simulink model "acc_with_sensor"  (R2021b)
settings: Solver=FixedStepAuto  StartTime=0.0  StopTime=206  FixedStep=0.0005  RelTol=1e-3
InitFcn:
  | G=9.81;
  | m=1660;
  | rw=0.325;
  | Caf=74070;
  | Car=58525;
  | Iz=2778.5;
  | d = 1.502;
  | lf =1.1135;
  | lr =1.5065;
  | L = 2.62;
  | kph2mps=1/3.6;
values from neighbouring files (symbols this model uses):
  Leftdis_PV_switch = 2    [acc_plot_backup.m]
  s_path = [0 1.10508939428 2.2141958029 3.32141571172 4.42705301151 5.53154548532 6.63517443471 7.73808041313 8.84055018688 9.94289959674 11.0453539299 12.1480581097 ... (1001 elements, 1001x1)]    [200_100radius.mat]    (also in LV_Clothoid_S_Turn_path.mat = [0 0.966832089581 1.93621320584 2.90214024471 3.86476766313 ; NEDC_path.mat = [0 0.414605943146 0.832514087334 1.25401518562 1.68216660344; Straight_East_into_curve.mat = [0 1.65770560069 3.32192925577 4.98420060507 6.64484613518 8; acc_plot_backup.m = Station_HV_m)
  X_path = [0 1.10508939428 2.2141958029 3.32141571172 4.42705301151 5.53154548532 6.63517443471 7.73808041313 8.84055018688 9.94289959674 11.0453539299 12.1480581097 ... (1001 elements, 1001x1)]    [200_100radius.mat]    (also in LV_Clothoid_S_Turn_path.mat = [-10 -9.03316791042 -8.06378679416 -7.09785975529 -6.1352323; NEDC_path.mat = [0 0.414605943146 0.832514087334 1.25401518562 1.68216660344; Straight_East_into_curve.mat = [0 1.65770560069 3.32192925577 4.98420060507 6.64484613518 8; acc_plot_backup.m = X_HV_m)
  Y_path = [0 -1.70364610795e-18 -7.41532896709e-18 1.46822109542e-17 4.74557362791e-17 6.12980216762e-17 9.25043977736e-17 1.24088240159e-16 1.5099156923e-16 1.7058517853e-16 1.90629227614e-16 2.09673434424e-16 ... (1001 elements, 1001x1)]    [200_100radius.mat]    (also in LV_Clothoid_S_Turn_path.mat = [0 -8.46153035536e-19 5.07382551045e-18 2.07356032218e-17 3.; NEDC_path.mat = [0 -3.50680326162e-18 -2.14111304971e-18 3.38197671014e-18 3; Straight_East_into_curve.mat = [0 1.29197709199e-18 2.81882429322e-18 3.49020462564e-17 6.7; acc_plot_backup.m = Y_HV_m)
undefined symbols (not defined in the file or in its folder): C_TICK_TIME_S, Cut_in_Secenary_flg, ENUM_ACCSTATE_DISABLED, ENUM_ACCSTATE_OFF, ENUM_ACCSTATE_STANDBY, FALSE, KVDI_ACCLongPressTime_ms, KVDI_ACCMaxActSpeed_kph, KVDI_ACCSetSpdIntial_kph, KVDI_ACCSpdLargeChange_kph, KVDI_LongPressConTime_ms, ONE_FLOAT, ONE_INT, raptor_xcp_function, T, TRUE, UseTTC_switch, ZERO_FLOAT, ZERO_INT
libraries: ADASLibrary x29, simulink x22, Raptor_lib x11, dspstat3 x6, simulink_extras x6, Solver_SF x1, mpclib x1
(part 3 of 9)

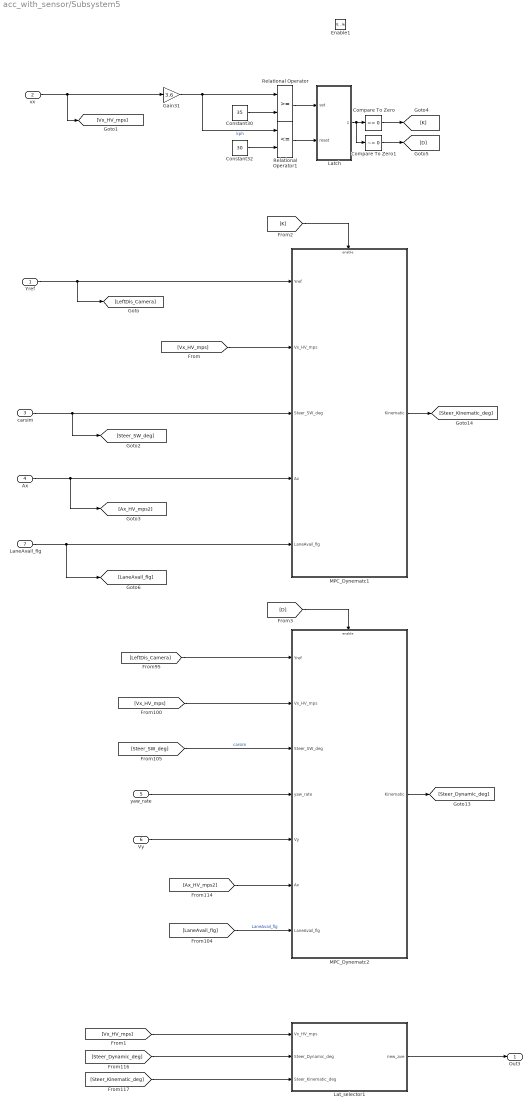
== system acc_with_sensor/Subsystem5 ==
  Yref : Inport
  vx : Inport  Port=2
  carsim : Inport  Port=3
  Ax : Inport  Port=4
  yaw_rate : Inport  Port=5
  Vy : Inport  Port=6
  LaneAvail_flg : Inport  Port=7
  Enable1 : EnablePort  StatesWhenEnabling=reset
  Compare To Zero : simulink/Logic and Bit Operations/Compare To Zero  relop===  OutDataTypeStr=boolean
  Compare To Zero1 : simulink/Logic and Bit Operations/Compare To Zero  relop=~=  OutDataTypeStr=boolean
  Constant30 : Constant  Value=35  SampleTime=-1
  Constant32 : Constant  Value=30  SampleTime=-1
  Gain31 : Gain  Gain=3.6
  Lat_selector1 : Subsystem
  Latch : Subsystem
  MPC_Dynematc1 : Subsystem
  MPC_Dynematc2 : Subsystem
  Relational Operator : RelationalOperator  OutDataTypeStr=boolean  RndMeth=Simplest
  Relational Operator1 : RelationalOperator  Operator=<=  OutDataTypeStr=boolean  RndMeth=Simplest
  Out3 : Outport
  wires:
  Yref/1 -> [LeftDis_Camera], MPC_Dynematc1/1(Yref)
  yaw_rate/1 -> MPC_Dynematc2/4(yaw_rate)
  carsim/1 -> [Steer_SW_deg], MPC_Dynematc1/3(Steer_SW_deg)
  [Steer_Dynamic_deg] -> Lat_selector1/2(Steer_Dynamic_deg)
  [Vx_HV_mps] -> MPC_Dynematc2/2(Vx_HV_mps)
  Vy/1 -> MPC_Dynematc2/5(Vy)
  Ax/1 -> [Ax_HV_mps2], MPC_Dynematc1/4(Ax)
  Lat_selector1/1(new_ave) -> Out3/1
  [Steer_Kinematic_deg] -> Lat_selector1/3(Steer_Kinematic_deg)
  MPC_Dynematc1/1(Kinematic) -> [Steer_Kinematic_deg]
  MPC_Dynematc2/1(Kinematic) -> [Steer_Dynamic_deg]
  [LeftDis_Camera] -> MPC_Dynematc2/1(Yref)
  [Steer_SW_deg] -> MPC_Dynematc2/3(Steer_SW_deg)  "carsim"
  [Ax_HV_mps2] -> MPC_Dynematc2/6(Ax)
  [Vx_HV_mps] -> Lat_selector1/1(Vx_HV_mps)
  Gain31/1 -> Relational Operator/1, Relational Operator1/1  "kph"
  Relational Operator/1 -> Latch/1(set)
  Relational Operator1/1 -> Latch/2(reset)
  Constant30/1 -> Relational Operator/2
  Constant32/1 -> Relational Operator1/2
  vx/1 -> [Vx_HV_mps], Gain31/1
  [Vx_HV_mps] -> MPC_Dynematc1/2(Vx_HV_mps)
  Latch/1(latched) -> Compare To Zero1/1, Compare To Zero/1
  Compare To Zero/1 -> [K]
  Compare To Zero1/1 -> [D]
  [K] -> MPC_Dynematc1/Enable
  [D] -> MPC_Dynematc2/Enable
  LaneAvail_flg/1 -> [LaneAvail_flg], MPC_Dynematc1/5(LaneAvail_flg)
  [LaneAvail_flg] -> MPC_Dynematc2/7(LaneAvail_flg)  "LaneAvail_flg"

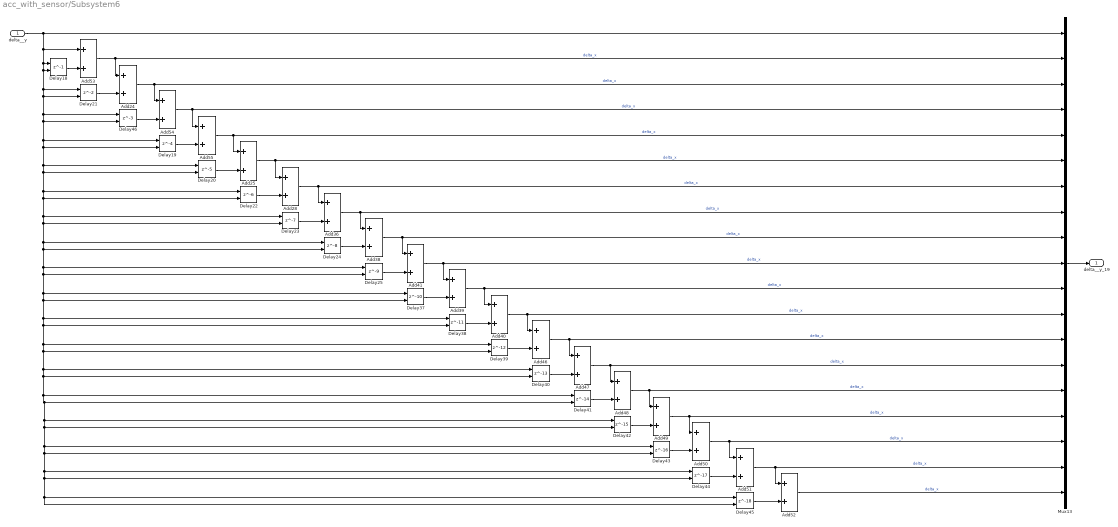
== system acc_with_sensor/Subsystem6 ==
  delta__y : Inport
  Add{24..25,28,36,38..41,46..55} (18 alike) : Sum
  Delay18 : Delay  DelayLength=1  InitialConditionSource=Input port
      settings: InputPortMap=u0,p4
  Delay19 : Delay  DelayLength=4  InitialConditionSource=Input port
      settings: InputPortMap=u0,p4
  Delay20 : Delay  DelayLength=5  InitialConditionSource=Input port
      settings: InputPortMap=u0,p4
  Delay21 : Delay  InitialConditionSource=Input port
      settings: InputPortMap=u0,p4
  Delay22 : Delay  DelayLength=6  InitialConditionSource=Input port
      settings: InputPortMap=u0,p4
  Delay23 : Delay  DelayLength=7  InitialConditionSource=Input port
      settings: InputPortMap=u0,p4
  Delay24 : Delay  DelayLength=8  InitialConditionSource=Input port
      settings: InputPortMap=u0,p4
  Delay25 : Delay  DelayLength=9  InitialConditionSource=Input port
      settings: InputPortMap=u0,p4
  Delay37 : Delay  DelayLength=10  InitialConditionSource=Input port
      settings: InputPortMap=u0,p4
  Delay38 : Delay  DelayLength=11  InitialConditionSource=Input port
      settings: InputPortMap=u0,p4
  Delay39 : Delay  DelayLength=12  InitialConditionSource=Input port
      settings: InputPortMap=u0,p4
  Delay40 : Delay  DelayLength=13  InitialConditionSource=Input port
      settings: InputPortMap=u0,p4
  Delay41 : Delay  DelayLength=14  InitialConditionSource=Input port
      settings: InputPortMap=u0,p4
  Delay42 : Delay  DelayLength=15  InitialConditionSource=Input port
      settings: InputPortMap=u0,p4
  Delay43 : Delay  DelayLength=16  InitialConditionSource=Input port
      settings: InputPortMap=u0,p4
  Delay44 : Delay  DelayLength=17  InitialConditionSource=Input port
      settings: InputPortMap=u0,p4
  Delay45 : Delay  DelayLength=18  InitialConditionSource=Input port
      settings: InputPortMap=u0,p4
  Delay46 : Delay  DelayLength=3  InitialConditionSource=Input port
      settings: InputPortMap=u0,p4
  Mux13 : Mux  Inputs=19
  delta__y_19 : Outport
  wires:
  Delay21/1 -> Add24/2
  delta__y/1 -> Mux13/1, Delay21/2, Delay46/1, Delay22/1, Delay25/2, Delay37/1, Delay39/2, Delay40/1, Delay41/1, Delay42/1, Delay42/2, Delay43/1, Delay44/1, Delay45/1, Delay45/2, Delay44/2, Delay43/2, Delay41/2, Delay40/2, Delay39/1, Delay38/2, Delay38/1, Delay37/2, Delay25/1, Delay24/2, Delay24/1, Delay23/2, Delay23/1, Delay22/2, Delay20/2, Delay20/1, Delay19/2, Delay19/1, Delay46/2, Delay21/1, Delay18/2, Delay18/1, Add53/1
  Delay22/1 -> Add28/2
  Add46/1 -> Mux13/13, Add47/1  "delta_x"
  Delay37/1 -> Add39/2
  Add39/1 -> Mux13/11, Add40/1  "delta_x"
  Delay38/1 -> Add40/2
  Add40/1 -> Mux13/12, Add46/1  "delta_x"
  Add38/1 -> Mux13/9, Add41/1  "delta_x"
  Add53/1 -> Mux13/2, Add24/1  "delta_x"
  Add55/1 -> Mux13/5, Add25/1  "delta_x"
  Add50/1 -> Add51/1, Mux13/17  "delta_x"
  Add47/1 -> Mux13/14, Add48/1  "delta_x"
  Delay39/1 -> Add46/2
  Delay40/1 -> Add47/2
  Mux13/1 -> delta__y_19/1
  Delay46/1 -> Add54/2
  Delay25/1 -> Add41/2
  Add52/1 -> Mux13/19  "delta_x"
  Add28/1 -> Mux13/7, Add36/1  "delta_x"
  Add36/1 -> Mux13/8, Add38/1  "delta_x"
  Delay23/1 -> Add36/2
  Delay20/1 -> Add25/2
  Delay42/1 -> Add49/2
  Delay44/1 -> Add51/2
  Delay18/1 -> Add53/2
  Add25/1 -> Mux13/6, Add28/1  "delta_x"
  Add41/1 -> Mux13/10, Add39/1  "delta_x"
  Add49/1 -> Add50/1, Mux13/16  "delta_x"
  Add51/1 -> Add52/1, Mux13/18  "delta_x"
  Delay19/1 -> Add55/2
  Add24/1 -> Mux13/3, Add54/1  "delta_x"
  Delay45/1 -> Add52/2
  Delay41/1 -> Add48/2
  Add54/1 -> Mux13/4, Add55/1  "delta_x"
  Delay24/1 -> Add38/2
  Delay43/1 -> Add50/2
  Add48/1 -> Mux13/15, Add49/1  "delta_x"

== system acc_with_sensor/Subsystem7 ==
  A : Inport
  B : Inport  Port=2
  C : Inport  Port=3
  Yref : Inport  Port=4
  x_state : Inport  Port=5
  u_old : Inport  Port=6
  Enable : EnablePort  StatesWhenEnabling=reset
  Constant104 : Constant  Value=Np  SampleTime=T
  Constant105 : Constant  Value=Nc  SampleTime=T
  Constant106 : Constant  Value=Q  SampleTime=T
  Constant107 : Constant  Value=R  SampleTime=T
  MPC_ACC4 : MATLAB Function  TreatAsAtomicUnit=on
  cmd : Outport
  wires:
  u_old/1 -> MPC_ACC4/10(u_old)
  Constant107/1 -> MPC_ACC4/9(Rs)
  Constant104/1 -> MPC_ACC4/6(Np)
  Constant106/1 -> MPC_ACC4/8(Qs)
  MPC_ACC4/1(u) -> cmd/1  "cmd"
  Constant105/1 -> MPC_ACC4/7(Nc)
  A/1 -> MPC_ACC4/1(A)
  C/1 -> MPC_ACC4/3(C)
  Yref/1 -> MPC_ACC4/4(Yref)
  B/1 -> MPC_ACC4/2(B)
  x_state/1 -> MPC_ACC4/5(x_state)

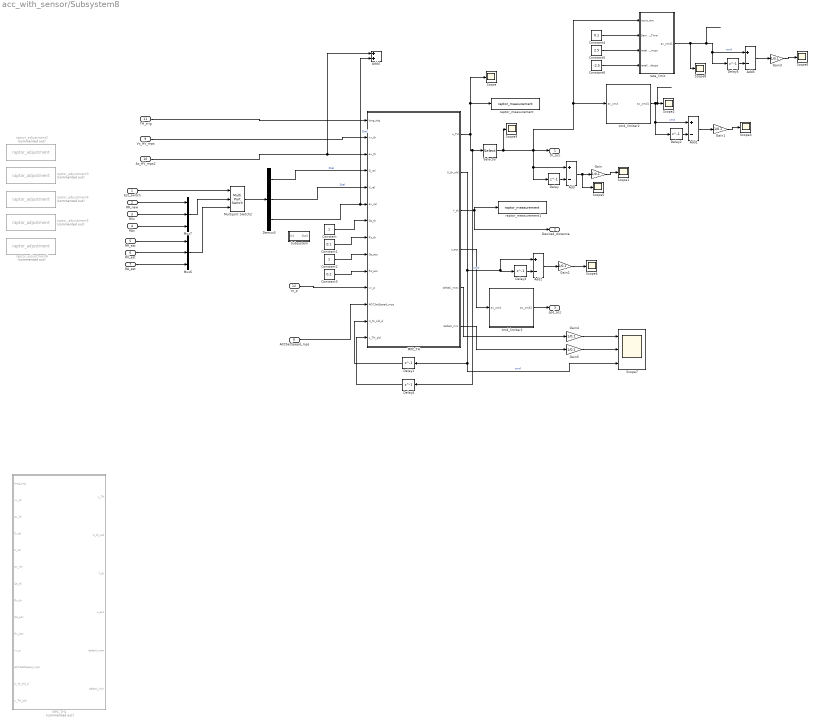
== system acc_with_sensor/Subsystem8 ==
  Est_switch : Inport
  RR_new : Inport  Port=2
  RVx : Inport  Port=3
  RAx : Inport  Port=4
  RR_est : Inport  Port=5
  RV_est : Inport  Port=6
  RA_est : Inport  Port=7
  ACCSetSpeed_mps : Inport  Port=8
  Vx_HV_mps : Inport  Port=9
  Ax_HV_mps2 : Inport  Port=10
  TH_trig : Inport  Port=11
  vx_p : Inport  Port=12
  Add{,1..3} (4 alike) : Sum  Inputs=+-
  Add4 : Sum
  Constant : Constant  SampleTime=T
  Constant1 : Constant  Value=0.1  SampleTime=T
  Constant2 : Constant  SampleTime=T
  Constant3 : Constant  Value=0.2  SampleTime=T
  Constant4 : Constant  Value=0.1  SampleTime=T
  Constant5 : Constant  Value=2.5  SampleTime=T
  Constant6 : Constant  Value=-2.5  SampleTime=T
  Delay{,2..3,5} (4 alike) : Delay  DelayLength=1
  Delay1 : Delay  DelayLength=1  SampleTime=T
  Delay4 : Delay  DelayLength=1  SampleTime=T
  Demux3 : Demux  Outputs=3
  Gain{,1..5} (6 alike) : Gain  Gain=1/0.1
  MPC_TH : MATLAB Function  TreatAsAtomicUnit=on
  MPC_TH1 : MATLAB Function  Commented=on  TreatAsAtomicUnit=on
  Multiport Switch2 : MultiPortSwitch  DataPortOrder=Zero-based contiguous  Inputs=2  DiagnosticForDefault=None  zeroidx=on
  Mux6 : Mux  Inputs=3
  Mux7 : Mux  Inputs=3
  Scope{,1..6,8..9} (9 alike) : Scope
  Scope7 : Scope  NumInputPorts=3
  Selector : Selector  InputPortWidth=3  IndexOptions=Index vector (dialog)  Indices=[1]  OutputSizes=1
  Subsystem : Subsystem
  cmd_limiter1 : Subsystem
  cmd_limiter2 : Subsystem
  raptor_adjustment2 : Raptor_lib/Data Storage/raptor_adjustment  Commented=on  paramName='Vx_th'  nameSource=Parameter  initValue=0.00  dataType=double  storage=Calibration  calDispType=Number  calEnum={'False', 'True'}  calGain=1.0  calOffset=0.0  calMax=inf  calMin=-inf  calFormat='-1'  calUnit=''  calHelp=''  calAccess=1  calFunction=raptor_xcp_function(gcb)  calDispHeaders=off  calColHeaders={'Col1' 'Col2' 'Col3'}  calRowHeaders={'Row1' 'Row2' 'Row3'}
      settings: SourceProductName=Raptor
  raptor_adjustment3 : Raptor_lib/Data Storage/raptor_adjustment  Commented=on  paramName='Ax_th'  nameSource=Parameter  initValue=0.00  dataType=double  storage=Calibration  calDispType=Number  calEnum={'False', 'True'}  calGain=1.0  calOffset=0.0  calMax=inf  calMin=-inf  calFormat='-1'  calUnit=''  calHelp=''  calAccess=1  calFunction=raptor_xcp_function(gcb)  calDispHeaders=off  calColHeaders={'Col1' 'Col2' 'Col3'}  calRowHeaders={'Row1' 'Row2' 'Row3'}
      settings: SourceProductName=Raptor
  raptor_adjustment4 : Raptor_lib/Data Storage/raptor_adjustment  Commented=on  paramName='D_rel'  nameSource=Parameter  initValue=1  dataType=double  storage=Calibration  calDispType=Number  calEnum={'False', 'True'}  calGain=1.0  calOffset=0.0  calMax=inf  calMin=-inf  calFormat='-1'  calUnit=''  calHelp=''  calAccess=1  calFunction=raptor_xcp_function(gcb)  calDispHeaders=off  calColHeaders={'Col1' 'Col2' 'Col3'}  calRowHeaders={'Row1' 'Row2' 'Row3'}
      settings: SourceProductName=Raptor
  raptor_adjustment5 : Raptor_lib/Data Storage/raptor_adjustment  Commented=on  paramName='V_rel'  nameSource=Parameter  initValue=1  dataType=double  storage=Calibration  calDispType=Number  calEnum={'False', 'True'}  calGain=1.0  calOffset=0.0  calMax=inf  calMin=-inf  calFormat='-1'  calUnit=''  calHelp=''  calAccess=1  calFunction=raptor_xcp_function(gcb)  calDispHeaders=off  calColHeaders={'Col1' 'Col2' 'Col3'}  calRowHeaders={'Row1' 'Row2' 'Row3'}
      settings: SourceProductName=Raptor
  raptor_adjustment6 : Raptor_lib/Data Storage/raptor_adjustment  Commented=on  paramName='ax_rel'  nameSource=Parameter  initValue=1  dataType=double  storage=Calibration  calDispType=Number  calEnum={'False', 'True'}  calGain=1.0  calOffset=0.0  calMax=inf  calMin=-inf  calFormat='-1'  calUnit=''  calHelp=''  calAccess=1  calFunction=raptor_xcp_function(gcb)  calDispHeaders=off  calColHeaders={'Col1' 'Col2' 'Col3'}  calRowHeaders={'Row1' 'Row2' 'Row3'}
      settings: SourceProductName=Raptor
  raptor_measurement : Raptor_lib/Data Storage/raptor_measurement  paramName='TH_acc'  nameSource=Parameter  calDispType=Number  calEnum={'False', 'True'}  calGain=1.0  calOffset=0.0  calMax=inf  calMin=-inf  calFormat='-1'  calUnit=''  calHelp=''  calAccess=1  calFunction=raptor_xcp_function(gcb)  calVisible=on
      settings: SourceProductName=Raptor
  raptor_measurement1 : Raptor_lib/Data Storage/raptor_measurement  paramName='Desired_distance'  nameSource=Parameter  calDispType=Number  calEnum={'False', 'True'}  calGain=1.0  calOffset=0.0  calMax=inf  calMin=-inf  calFormat='-1'  calUnit=''  calHelp=''  calAccess=1  calFunction=raptor_xcp_function(gcb)  calVisible=on
      settings: SourceProductName=Raptor
  rate_limit : Subsystem
  th_acc : Outport
  Desired_distance : Outport  Port=2
  spd_acc : Outport  Port=3
  wires:
  Demux3/3 -> Add4/2, MPC_TH/6(ax_rel)  "Drel"
  Demux3/2 -> MPC_TH/5(V_rel)  "Drel"
  ACCSetSpeed_mps/1 -> MPC_TH/12(ACCSetSpeed_mps)
  Est_switch/1 -> Multiport Switch2/1
  RA_est/1 -> Mux6/3
  RVx/1 -> Mux7/2
  Constant/1 -> MPC_TH/7(Qs_th)
  Vx_HV_mps/1 -> MPC_TH/2(vx_th)
  MPC_TH/3(Y_th) -> Desired_distance/1, raptor_measurement1/1
  Mux6/1 -> Multiport Switch2/3
  Mux7/1 -> Multiport Switch2/2
  Ax_HV_mps2/1 -> Add4/1, MPC_TH/3(ax_th)
  RAx/1 -> Mux7/3
  RR_est/1 -> Mux6/1
  Constant1/1 -> MPC_TH/8(Rs_th)
  Demux3/1 -> MPC_TH/4(D_rel)  "Drel"
  TH_trig/1 -> MPC_TH/1(long_trig)
  RR_new/1 -> Mux7/1
  RV_est/1 -> Mux6/2
  MPC_TH/1(u_TH) -> Delay4/1, Selector/1, raptor_measurement/1, Scope/1  "cmd"
  Multiport Switch2/1 -> Demux3/1
  Constant2/1 -> MPC_TH/9(Qs_acc)
  Constant3/1 -> MPC_TH/10(Rs_acc)
  MPC_TH/4(u_acc) -> cmd_limiter1/1(ax_cmd)
  cmd_limiter1/1(ax_cmd1) -> spd_acc/1
  vx_p/1 -> MPC_TH/11(vx_p)
  Delay/1 -> Add/2
  Add/1 -> Scope5/1, Gain/1
  Gain/1 -> Scope1/1
  Delay1/1 -> MPC_TH/13(U_th_old_d)
  Gain1/1 -> Scope3/1
  Add1/1 -> Gain1/1
  Delay2/1 -> Add1/2
  cmd_limiter2/1(ax_cmd1) -> Add1/1, Delay2/1, Scope2/1  "cmd"
  Gain2/1 -> Scope4/1
  Add2/1 -> Gain2/1
  Delay3/1 -> Add2/2
  MPC_TH/2(U_th_old) -> Add2/1, Delay3/1, Delay1/1, Scope7/3  "cmd"
  Delay4/1 -> MPC_TH/14(u_TH_old)
  Constant5/1 -> rate_limit/3(ratelimt_incps)
  Constant4/1 -> rate_limit/2(Sample_Time)
  Constant6/1 -> rate_limit/4(ratelimt_decps)
  rate_limit/1(ax_cmd1) -> Scope8/1, Delay5/1, Add3/1  "cmd"
  Delay5/1 -> Add3/2
  Add3/1 -> Gain3/1
  Gain3/1 -> Scope6/1
  MPC_TH/5(deltaU_max) -> Gain4/1
  MPC_TH/6(deltaU_min) -> Gain5/1
  Gain4/1 -> Scope7/1
  Gain5/1 -> Scope7/2
  Selector/1 -> Scope9/1, th_acc/1, rate_limit/1(input_raw), cmd_limiter2/1(ax_cmd), Delay/1, Add/1

== system acc_with_sensor/V_rel Estimation ==
  cut_in_flg : Inport
  a_c : Inport  Port=2
  S_rel : Inport  Port=3
  initial_value : Inport  Port=4
  Enable : EnablePort  StatesWhenEnabling=reset
  Add3 : Sum  Inputs=-+
  Delay1 : Delay  DelayLength=1  InitialConditionSource=Input port  SampleTime=T
      settings: InputPortMap=u0,p4
  Kalman filter : Subsystem
  sample time : Gain  Gain=1/0.1
  s_rel : Outport
  v_rel : Outport  Port=2
  a_rel : Outport  Port=3
  wires:
  S_rel/1 -> Kalman filter/3(S_rel)
  Kalman filter/1(s_rel) -> s_rel/1
  Add3/1 -> sample time/1
  Delay1/1 -> Add3/1
  a_c/1 -> Delay1/1, Delay1/2, Add3/2
  Kalman filter/2(v_rel) -> v_rel/1
  sample time/1 -> Kalman filter/2(Jerk)  "Jerk"
  Kalman filter/3(a_rel) -> a_rel/1
  initial_value/1 -> Kalman filter/4(initial_value)
  cut_in_flg/1 -> Kalman filter/1(cut_in_flg)

== system acc_with_sensor/cmd_limiter1 ==
  ax_cmd : Inport
  Constant : Constant  Value=0.1  SampleTime=T
  Constant1 : Constant  Value=2.5  SampleTime=T
  Constant2 : Constant  Value=-2.5  SampleTime=T
  Saturation : Saturate  UpperLimit=2  LowerLimit=-2
  rate_limit : Subsystem
  ax_cmd1 : Outport
  wires:
  Saturation/1 -> rate_limit/1(input_raw)
  Constant2/1 -> rate_limit/4(ratelimt_decps)
  Constant1/1 -> rate_limit/3(ratelimt_incps)
  ax_cmd/1 -> Saturation/1
  Constant/1 -> rate_limit/2(Sample_Time)
  rate_limit/1(ax_cmd1) -> ax_cmd1/1

== system acc_with_sensor/cmd_limiter11 ==
  ax_cmd : Inport
  Constant : Constant  Value=0.1  SampleTime=T
  Constant1 : Constant  Value=2.5  SampleTime=T
  Constant2 : Constant  Value=-2.5  SampleTime=T
  Constant3 : Constant  Value=2  SampleTime=T
  Constant4 : Constant  Value=-2  SampleTime=T
  Limit : ADASLibrary/Limit  SystemSampleTime=-1  VariantActivationTime=update diagram  Latency=0  AutoFrameSizeCalculation=off
      settings: SourceProductName=ADASLibrary
  rate_limit : Subsystem
  ax_cmd1 : Outport
  wires:
  rate_limit/1(ax_cmd1) -> ax_cmd1/1
  Constant/1 -> rate_limit/2(Sample_Time)
  ax_cmd/1 -> Limit/1
  Constant1/1 -> rate_limit/3(ratelimt_incps)
  Constant2/1 -> rate_limit/4(ratelimt_decps)
  Limit/1 -> rate_limit/1(input_raw)
  Constant3/1 -> Limit/2
  Constant4/1 -> Limit/3

== system acc_with_sensor/cmd_limiter2 ==
  ax_cmd : Inport
  Constant : Constant  Value=0.1  SampleTime=T
  Constant1 : Constant  Value=2.5  SampleTime=T
  Constant2 : Constant  Value=-2.5  SampleTime=T
  Constant3 : Constant  Value=2  SampleTime=T
  Constant4 : Constant  Value=-2  SampleTime=T
  Limit : ADASLibrary/Limit  SystemSampleTime=-1  VariantActivationTime=update diagram  Latency=0  AutoFrameSizeCalculation=off
      settings: SourceProductName=ADASLibrary
  rate_limit : Subsystem
  ax_cmd1 : Outport
  wires:
  Constant4/1 -> Limit/3
  Constant3/1 -> Limit/2
  Limit/1 -> rate_limit/1(input_raw)
  Constant2/1 -> rate_limit/4(ratelimt_decps)
  Constant1/1 -> rate_limit/3(ratelimt_incps)
  ax_cmd/1 -> Limit/1
  Constant/1 -> rate_limit/2(Sample_Time)
  rate_limit/1(ax_cmd1) -> ax_cmd1/1

== system acc_with_sensor/cmd_limiter3 ==
  ax_cmd : Inport
  Constant : Constant  Value=0.1  SampleTime=T
  Constant1 : Constant  Value=2.5  SampleTime=T
  Constant2 : Constant  Value=-2.5  SampleTime=T
  Constant3 : Constant  Value=2  SampleTime=T
  Constant4 : Constant  Value=-2  SampleTime=T
  Limit : ADASLibrary/Limit  SystemSampleTime=-1  VariantActivationTime=update diagram  Latency=0  AutoFrameSizeCalculation=off
      settings: SourceProductName=ADASLibrary
  rate_limit : Subsystem
  ax_cmd1 : Outport
  wires:
  Constant4/1 -> Limit/3
  Constant3/1 -> Limit/2
  Limit/1 -> rate_limit/1(input_raw)
  Constant2/1 -> rate_limit/4(ratelimt_decps)
  Constant1/1 -> rate_limit/3(ratelimt_incps)
  ax_cmd/1 -> Limit/1
  Constant/1 -> rate_limit/2(Sample_Time)
  rate_limit/1(ax_cmd1) -> ax_cmd1/1

== system acc_with_sensor/cmd_limiter4 ==
  ax_cmd : Inport
  Constant : Constant  Value=0.1  SampleTime=T
  Constant1 : Constant  Value=2.5  SampleTime=T
  Constant2 : Constant  Value=-2.5  SampleTime=T
  Saturation : Saturate  UpperLimit=2  LowerLimit=-2
  rate_limit : Subsystem
  ax_cmd1 : Outport
  wires:
  rate_limit/1(ax_cmd1) -> ax_cmd1/1
  Constant/1 -> rate_limit/2(Sample_Time)
  ax_cmd/1 -> Saturation/1
  Constant1/1 -> rate_limit/3(ratelimt_incps)
  Constant2/1 -> rate_limit/4(ratelimt_decps)
  Saturation/1 -> rate_limit/1(input_raw)

== system acc_with_sensor/cmd_limiter9 ==
  ax_cmd : Inport
  Constant : Constant  Value=0.1  SampleTime=T
  Constant1 : Constant  Value=2.5  SampleTime=T
  Constant2 : Constant  Value=-2.5  SampleTime=T
  Saturation : Saturate  UpperLimit=2  LowerLimit=-2
  rate_limit : Subsystem
  ax_cmd1 : Outport
  wires:
  rate_limit/1(ax_cmd1) -> ax_cmd1/1
  Constant/1 -> rate_limit/2(Sample_Time)
  ax_cmd/1 -> Saturation/1
  Constant1/1 -> rate_limit/3(ratelimt_incps)
  Constant2/1 -> rate_limit/4(ratelimt_decps)
  Saturation/1 -> rate_limit/1(input_raw)

== system acc_with_sensor/divide ==
  dividend : Inport
  divisor : Inport  Port=2
  default_value : Inport  Port=3
  Divide : Product  Inputs=*/
  Interval Test : simulink/Logic and Bit Operations/Interval Test  IntervalClosedRight=on  uplimit=5/3.6  IntervalClosedLeft=on  lowlimit=-1  OutDataTypeStr=boolean
  Logical Operator : Logic  Operator=NOT  Inputs=1  AllPortsSameDT=off  OutDataTypeStr=boolean
  Scope : Scope
  Switch : Switch  Criteria=u2 ~= 0  Threshold=0.5
  quotient : Outport
  wires:
  Logical Operator/1 -> Switch/2
  default_value/1 -> Switch/3  "default_value"
  Interval Test/1 -> Scope/1, Logical Operator/1
  Switch/1 -> quotient/1
  Divide/1 -> Switch/1
  divisor/1 -> Interval Test/1, Divide/2  "divisor"
  dividend/1 -> Divide/1  "dividend"

== system acc_with_sensor/divide2 ==
  dividend : Inport
  divisor : Inport  Port=2
  default_value : Inport  Port=3
  Divide : Product  Inputs=*/
  Interval Test : simulink/Logic and Bit Operations/Interval Test  IntervalClosedRight=on  uplimit=15/3.6  IntervalClosedLeft=on  lowlimit=-1  OutDataTypeStr=boolean
  Logical Operator : Logic  Operator=NOT  Inputs=1  AllPortsSameDT=off  OutDataTypeStr=boolean
  Scope : Scope
  Switch : Switch  Criteria=u2 ~= 0  Threshold=0.5
  quotient : Outport
  wires:
  dividend/1 -> Divide/1  "dividend"
  divisor/1 -> Divide/2, Interval Test/1  "divisor"
  Divide/1 -> Switch/1
  Switch/1 -> quotient/1
  Interval Test/1 -> Logical Operator/1, Scope/1
  default_value/1 -> Switch/3  "default_value"
  Logical Operator/1 -> Switch/2

== system acc_with_sensor/divide3 ==
  dividend : Inport
  divisor : Inport  Port=2
  default_value : Inport  Port=3
  Divide : Product  Inputs=*/
  Interval Test : simulink/Logic and Bit Operations/Interval Test  IntervalClosedRight=on  uplimit=-0.1  IntervalClosedLeft=on  lowlimit=-inf  OutDataTypeStr=boolean
  Logical Operator : Logic  Operator=NOT  Inputs=1  AllPortsSameDT=off  OutDataTypeStr=boolean
  Scope : Scope
  Switch : Switch  Criteria=u2 ~= 0  Threshold=0.5
  quotient : Outport
  wires:
  dividend/1 -> Divide/1  "dividend"
  divisor/1 -> Divide/2, Interval Test/1  "divisor"
  Divide/1 -> Switch/1
  Switch/1 -> quotient/1
  Interval Test/1 -> Logical Operator/1, Scope/1
  default_value/1 -> Switch/3  "default_value"
  Logical Operator/1 -> Switch/2

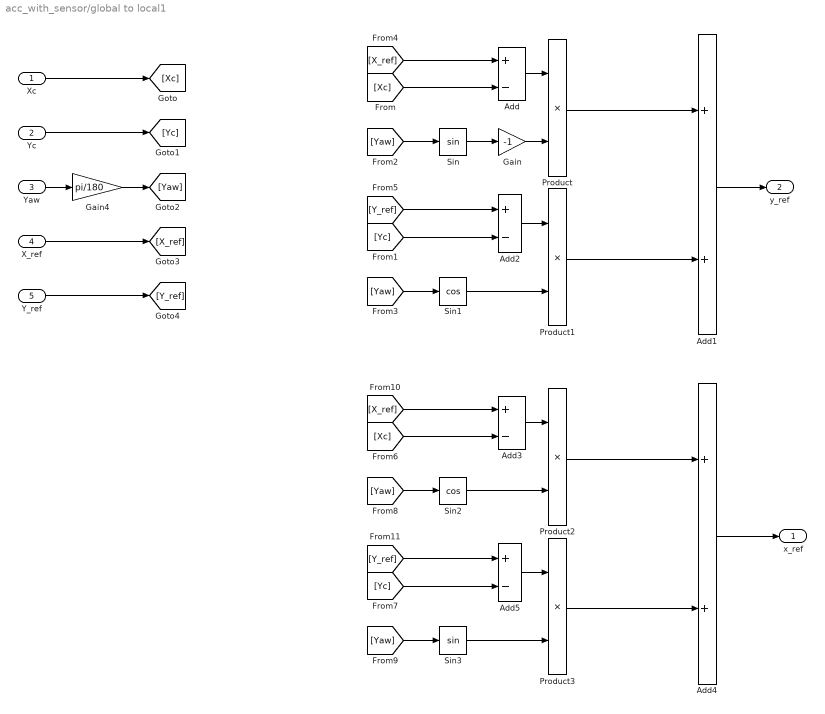
== system acc_with_sensor/global to local1 ==
  Xc : Inport
  Yc : Inport  Port=2
  Yaw : Inport  Port=3
  X_ref : Inport  Port=4
  Y_ref : Inport  Port=5
  Add{,2..3,5} (4 alike) : Sum  Inputs=+-
  Add1 : Sum
  Add4 : Sum
  Gain : Gain  Gain=-1
  Gain4 : Gain  Gain=pi/180
  Product{,1..3} (4 alike) : Product
  Sin : Trigonometry
  Sin1 : Trigonometry  Operator=cos
  Sin2 : Trigonometry  Operator=cos
  Sin3 : Trigonometry
  x_ref : Outport
  y_ref : Outport  Port=2
  wires:
  [X_ref] -> Add3/1
  [Y_ref] -> Add5/1
  Sin2/1 -> Product2/2
  Add3/1 -> Product2/1
  Product2/1 -> Add4/1
  Sin3/1 -> Product3/2
  Add5/1 -> Product3/1
  Product3/1 -> Add4/2
  Add4/1 -> x_ref/1
  [Yaw] -> Sin2/1
  [Yc] -> Add5/2
  [Xc] -> Add3/2
  [Yaw] -> Sin3/1
  Gain4/1 -> [Yaw]
  Y_ref/1 -> [Y_ref]
  X_ref/1 -> [X_ref]
  [Yaw] -> Sin1/1
  Yaw/1 -> Gain4/1
  Yc/1 -> [Yc]
  Xc/1 -> [Xc]
  [Xc] -> Add/2
  [Yc] -> Add2/2
  [Yaw] -> Sin/1
  Add1/1 -> y_ref/1
  Product1/1 -> Add1/2
  Add2/1 -> Product1/1
  Sin1/1 -> Product1/2
  Product/1 -> Add1/1
  Add/1 -> Product/1
  Gain/1 -> Product/2
  Sin/1 -> Gain/1
  [Y_ref] -> Add2/1
  [X_ref] -> Add/1

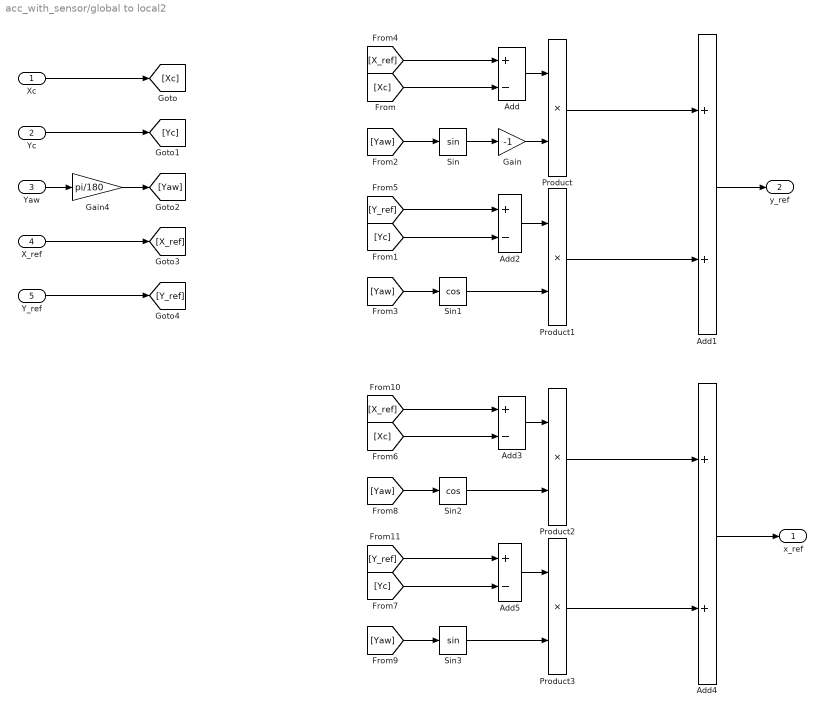
== system acc_with_sensor/global to local2 ==
  Xc : Inport
  Yc : Inport  Port=2
  Yaw : Inport  Port=3
  X_ref : Inport  Port=4
  Y_ref : Inport  Port=5
  Add{,2..3,5} (4 alike) : Sum  Inputs=+-
  Add1 : Sum
  Add4 : Sum
  Gain : Gain  Gain=-1
  Gain4 : Gain  Gain=pi/180
  Product{,1..3} (4 alike) : Product
  Sin : Trigonometry
  Sin1 : Trigonometry  Operator=cos
  Sin2 : Trigonometry  Operator=cos
  Sin3 : Trigonometry
  x_ref : Outport
  y_ref : Outport  Port=2
  wires:
  [X_ref] -> Add3/1
  [Y_ref] -> Add5/1
  Sin2/1 -> Product2/2
  Add3/1 -> Product2/1
  Product2/1 -> Add4/1
  Sin3/1 -> Product3/2
  Add5/1 -> Product3/1
  Product3/1 -> Add4/2
  Add4/1 -> x_ref/1
  [Yaw] -> Sin2/1
  [Yc] -> Add5/2
  [Xc] -> Add3/2
  [Yaw] -> Sin3/1
  Gain4/1 -> [Yaw]
  Y_ref/1 -> [Y_ref]
  X_ref/1 -> [X_ref]
  [Yaw] -> Sin1/1
  Yaw/1 -> Gain4/1
  Yc/1 -> [Yc]
  Xc/1 -> [Xc]
  [Xc] -> Add/2
  [Yc] -> Add2/2
  [Yaw] -> Sin/1
  Add1/1 -> y_ref/1
  Product1/1 -> Add1/2
  Add2/1 -> Product1/1
  Sin1/1 -> Product1/2
  Product/1 -> Add1/1
  Add/1 -> Product/1
  Gain/1 -> Product/2
  Sin/1 -> Gain/1
  [Y_ref] -> Add2/1
  [X_ref] -> Add/1

== system acc_with_sensor/global to local3 ==
  Xc : Inport
  Yc : Inport  Port=2
  Yaw : Inport  Port=3
  X_ref : Inport  Port=4
  Y_ref : Inport  Port=5
  Add : Sum  Inputs=+-
  Add1 : Sum
  Add2 : Sum  Inputs=+-
  Gain : Gain  Gain=-1
  Gain4 : Gain  Gain=pi/180
  Product : Product
  Product1 : Product
  Sin : Trigonometry
  Sin1 : Trigonometry  Operator=cos
  y_path_ref10 : Outport
  wires:
  Gain4/1 -> [Yaw]
  Y_ref/1 -> [Y_ref]
  X_ref/1 -> [X_ref]
  [Yaw] -> Sin1/1
  Yaw/1 -> Gain4/1
  Yc/1 -> [Yc]
  Xc/1 -> [Xc]
  [Xc] -> Add/2
  [Yc] -> Add2/2
  [Yaw] -> Sin/1
  Add1/1 -> y_path_ref10/1
  Product1/1 -> Add1/2
  Add2/1 -> Product1/1
  Sin1/1 -> Product1/2
  Product/1 -> Add1/1
  Add/1 -> Product/1
  Gain/1 -> Product/2
  Sin/1 -> Gain/1
  [Y_ref] -> Add2/1
  [X_ref] -> Add/1

== system acc_with_sensor/preview ==
  In1 : Inport
  In2 : Inport  Port=2
  Add9 : Sum
  Constant20 : Constant  Value=s_path
  Constant21 : Constant  Value=X_path
  Constant22 : Constant  Value=s_path
  Constant23 : Constant  Value=Y_path
  Constant49 : Constant  Value=[1:10]'
  Constant51 : Constant  Value=0.1
  Demux4 : Demux  Outputs=[1 9]
  Demux5 : Demux  Outputs=[1 9]
  Lookup Table Dynamic : simulink/Lookup Tables/Lookup Table Dynamic  LookUpMeth=Interpolation-Use End Values  OutDataType=fixdt('double')  OutScaling=[]  OutputDataTypeScalingMode=Specify via dialog  OutDataTypeStr=double  DoSatur=off
  Lookup Table Dynamic1 : simulink/Lookup Tables/Lookup Table Dynamic  LookUpMeth=Interpolation-Use End Values  OutDataType=fixdt('double')  OutScaling=[]  OutputDataTypeScalingMode=Specify via dialog  OutDataTypeStr=double  DoSatur=off
  Product1 : Product
  Product10 : Product
  Scope7 : Scope
  Terminator : Terminator
  Terminator1 : Terminator
  To Workspace27 : ToWorkspace  VariableName=X_ref  SampleTime=-1
  To Workspace28 : ToWorkspace  VariableName=Y_ref  SampleTime=-1
  X_ref : Outport
  Y_ref : Outport  Port=2
  wires:
  Constant23/1 -> Lookup Table Dynamic1/3
  Product10/1 -> Add9/2
  Product1/1 -> Product10/2
  Constant22/1 -> Lookup Table Dynamic1/2
  Constant20/1 -> Lookup Table Dynamic/2
  Constant21/1 -> Lookup Table Dynamic/3
  Lookup Table Dynamic1/1 -> Y_ref/1, Demux5/1
  Demux5/1 -> To Workspace28/1
  In1/1 -> Add9/1
  Lookup Table Dynamic/1 -> X_ref/1, Demux4/1
  In2/1 -> Product10/1
  Constant51/1 -> Product1/2
  Add9/1 -> Lookup Table Dynamic1/1, Scope7/1, Lookup Table Dynamic/1
  Constant49/1 -> Product1/1
  Demux4/1 -> To Workspace27/1
  Demux5/2 -> Terminator1/1
  Demux4/2 -> Terminator/1

== system acc_with_sensor/record_delta_x ==
  delta_x : Inport
  Add{5,7..8,18..19,21..23} (8 alike) : Sum
  Delay1 : Delay  DelayLength=1  InitialConditionSource=Input port
      settings: InputPortMap=u0,p4
  Delay12 : Delay  DelayLength=4  InitialConditionSource=Input port
      settings: InputPortMap=u0,p4
  Delay13 : Delay  DelayLength=5  InitialConditionSource=Input port
      settings: InputPortMap=u0,p4
  Delay14 : Delay  InitialConditionSource=Input port
      settings: InputPortMap=u0,p4
  Delay15 : Delay  DelayLength=6  InitialConditionSource=Input port
      settings: InputPortMap=u0,p4
  Delay16 : Delay  DelayLength=7  InitialConditionSource=Input port
      settings: InputPortMap=u0,p4
  Delay17 : Delay  DelayLength=8  InitialConditionSource=Input port
      settings: InputPortMap=u0,p4
  Delay9 : Delay  DelayLength=3  InitialConditionSource=Input port
      settings: InputPortMap=u0,p4
  Mux12 : Mux  Inputs=9
  Scope : Scope
  delta_x_19 : Outport
  wires:
  Add19/1 -> Mux12/6, Add21/1  "delta_x"
  Delay13/1 -> Add19/2
  delta_x/1 -> Delay14/2, Delay9/1, Delay15/1, Delay17/2, Delay17/1, Delay16/2, Delay16/1, Delay15/2, Delay13/2, Delay13/1, Delay12/2, Delay12/1, Delay9/2, Delay14/1, Delay1/2, Delay1/1, Add5/1, Mux12/1
  Add5/1 -> Mux12/2, Add18/1  "delta_x"
  Add18/1 -> Mux12/3, Add7/1  "delta_x"
  Delay1/1 -> Add5/2
  Add23/1 -> Mux12/9  "delta_x"
  Delay9/1 -> Add7/2
  Mux12/1 -> Scope/1, delta_x_19/1
  Delay14/1 -> Add18/2
  Add21/1 -> Mux12/7, Add22/1  "delta_x"
  Delay17/1 -> Add23/2
  Delay15/1 -> Add21/2
  Add8/1 -> Mux12/5, Add19/1  "delta_x"
  Delay16/1 -> Add22/2
  Add22/1 -> Add23/1, Mux12/8  "delta_x"
  Delay12/1 -> Add8/2
  Add7/1 -> Mux12/4, Add8/1  "delta_x"

== system acc_with_sensor/record_delta_x1 ==
  delta_x : Inport
  Add{3,5,7..8,18..19,21..23,27,29..31,37,42..45} (18 alike) : Sum
  Delay1 : Delay  DelayLength=1  InitialConditionSource=Input port
      settings: InputPortMap=u0,p4
  Delay12 : Delay  DelayLength=4  InitialConditionSource=Input port
      settings: InputPortMap=u0,p4
  Delay13 : Delay  DelayLength=5  InitialConditionSource=Input port
      settings: InputPortMap=u0,p4
  Delay14 : Delay  InitialConditionSource=Input port
      settings: InputPortMap=u0,p4
  Delay15 : Delay  DelayLength=6  InitialConditionSource=Input port
      settings: InputPortMap=u0,p4
  Delay16 : Delay  DelayLength=7  InitialConditionSource=Input port
      settings: InputPortMap=u0,p4
  Delay17 : Delay  DelayLength=8  InitialConditionSource=Input port
      settings: InputPortMap=u0,p4
  Delay27 : Delay  DelayLength=9  InitialConditionSource=Input port
      settings: InputPortMap=u0,p4
  Delay28 : Delay  DelayLength=10  InitialConditionSource=Input port
      settings: InputPortMap=u0,p4
  Delay29 : Delay  DelayLength=11  InitialConditionSource=Input port
      settings: InputPortMap=u0,p4
  Delay30 : Delay  DelayLength=12  InitialConditionSource=Input port
      settings: InputPortMap=u0,p4
  Delay31 : Delay  DelayLength=13  InitialConditionSource=Input port
      settings: InputPortMap=u0,p4
  Delay32 : Delay  DelayLength=14  InitialConditionSource=Input port
      settings: InputPortMap=u0,p4
  Delay33 : Delay  DelayLength=15  InitialConditionSource=Input port
      settings: InputPortMap=u0,p4
  Delay34 : Delay  DelayLength=16  InitialConditionSource=Input port
      settings: InputPortMap=u0,p4
  Delay35 : Delay  DelayLength=17  InitialConditionSource=Input port
      settings: InputPortMap=u0,p4
  Delay36 : Delay  DelayLength=18  InitialConditionSource=Input port
      settings: InputPortMap=u0,p4
  Delay9 : Delay  DelayLength=3  InitialConditionSource=Input port
      settings: InputPortMap=u0,p4
  Mux12 : Mux  Inputs=19
  delta_x_19 : Outport
  wires:
  Add19/1 -> Mux12/6, Add21/1  "delta_x"
  Delay13/1 -> Add19/2
  Add44/1 -> Add45/1, Mux12/18  "delta_x"
  delta_x/1 -> Mux12/1, Delay14/2, Delay9/1, Delay15/1, Delay27/2, Delay28/1, Delay30/2, Delay31/1, Delay32/1, Delay33/1, Delay33/2, Delay34/1, Delay35/1, Delay36/1, Delay36/2, Delay35/2, Delay34/2, Delay32/2, Delay31/2, Delay30/1, Delay29/2, Delay29/1, Delay28/2, Delay27/1, Delay17/2, Delay17/1, Delay16/2, Delay16/1, Delay15/2, Delay13/2, Delay13/1, Delay12/2, Delay12/1, Delay9/2, Delay14/1, Delay1/2, Delay1/1, Add5/1
  Add29/1 -> Mux12/12, Add30/1  "delta_x"
  Add5/1 -> Mux12/2, Add18/1  "delta_x"
  Add18/1 -> Mux12/3, Add7/1  "delta_x"
  Delay29/1 -> Add29/2
  Delay1/1 -> Add5/2
  Add31/1 -> Mux12/14, Add37/1  "delta_x"
  Delay33/1 -> Add42/2
  Add23/1 -> Mux12/9, Add3/1  "delta_x"
  Delay9/1 -> Add7/2
  Add42/1 -> Add43/1, Mux12/16  "delta_x"
  Mux12/1 -> delta_x_19/1
  Delay14/1 -> Add18/2
  Add21/1 -> Mux12/7, Add22/1  "delta_x"
  Add30/1 -> Mux12/13, Add31/1  "delta_x"
  Delay34/1 -> Add43/2
  Delay17/1 -> Add23/2
  Delay27/1 -> Add3/2
  Add45/1 -> Mux12/19  "delta_x"
  Delay31/1 -> Add31/2
  Add43/1 -> Add44/1, Mux12/17  "delta_x"
  Delay15/1 -> Add21/2
  Add8/1 -> Mux12/5, Add19/1  "delta_x"
  Delay32/1 -> Add37/2
  Delay35/1 -> Add44/2
  Delay36/1 -> Add45/2
  Add27/1 -> Mux12/11, Add29/1  "delta_x"
  Add3/1 -> Mux12/10, Add27/1  "delta_x"
  Delay28/1 -> Add27/2
  Delay16/1 -> Add22/2
  Add22/1 -> Mux12/8, Add23/1  "delta_x"
  Delay30/1 -> Add30/2
  Add37/1 -> Mux12/15, Add42/1  "delta_x"
  Delay12/1 -> Add8/2
  Add7/1 -> Mux12/4, Add8/1  "delta_x"

== system acc_with_sensor/record_delta_yaw ==
  delta_yaw : Inport
  Add78 : Sum  Inputs=+-
  Delay68 : Delay  DelayLength=1  InitialConditionSource=Input port
      settings: InputPortMap=u0,p4
  Delay69 : Delay  InitialConditionSource=Input port
      settings: InputPortMap=u0,p4
  Delay70 : Delay  DelayLength=3  InitialConditionSource=Input port
      settings: InputPortMap=u0,p4
  Delay71 : Delay  DelayLength=4  InitialConditionSource=Input port
      settings: InputPortMap=u0,p4
  Delay72 : Delay  DelayLength=5  InitialConditionSource=Input port
      settings: InputPortMap=u0,p4
  Delay73 : Delay  DelayLength=6  InitialConditionSource=Input port
      settings: InputPortMap=u0,p4
  Delay74 : Delay  DelayLength=7  InitialConditionSource=Input port
      settings: InputPortMap=u0,p4
  Delay75 : Delay  DelayLength=8  InitialConditionSource=Input port
      settings: InputPortMap=u0,p4
  Delay76 : Delay  DelayLength=9  InitialConditionSource=Input port
      settings: InputPortMap=u0,p4
  Mux18 : Mux  Inputs=9
  delta_yaw_19 : Outport
  wires:
  Delay72/1 -> Mux18/5
  Delay73/1 -> Mux18/6
  Delay71/1 -> Mux18/4
  Delay68/1 -> Mux18/1
  Delay76/1 -> Mux18/9
  delta_yaw/1 -> Delay68/1, Delay68/2, Delay76/2, Delay76/1, Delay75/2, Delay75/1, Delay74/2, Delay74/1, Delay73/2, Delay73/1, Delay72/2, Delay72/1, Delay71/2, Delay71/1, Delay70/2, Delay70/1, Delay69/2, Delay69/1, Add78/1
  Delay75/1 -> Mux18/8
  Delay69/1 -> Mux18/2
  Delay70/1 -> Mux18/3
  Delay74/1 -> Mux18/7
  Mux18/1 -> Add78/2
  Add78/1 -> delta_yaw_19/1

== system acc_with_sensor/record_delta_yaw1 ==
  delta_yaw : Inport
  Add78 : Sum  Inputs=+-
  Delay68 : Delay  DelayLength=1  InitialConditionSource=Input port
      settings: InputPortMap=u0,p4
  Delay69 : Delay  InitialConditionSource=Input port
      settings: InputPortMap=u0,p4
  Delay70 : Delay  DelayLength=3  InitialConditionSource=Input port
      settings: InputPortMap=u0,p4
  Delay71 : Delay  DelayLength=4  InitialConditionSource=Input port
      settings: InputPortMap=u0,p4
  Delay72 : Delay  DelayLength=5  InitialConditionSource=Input port
      settings: InputPortMap=u0,p4
  Delay73 : Delay  DelayLength=6  InitialConditionSource=Input port
      settings: InputPortMap=u0,p4
  Delay74 : Delay  DelayLength=7  InitialConditionSource=Input port
      settings: InputPortMap=u0,p4
  Delay75 : Delay  DelayLength=8  InitialConditionSource=Input port
      settings: InputPortMap=u0,p4
  Delay76 : Delay  DelayLength=9  InitialConditionSource=Input port
      settings: InputPortMap=u0,p4
  Delay77 : Delay  DelayLength=10  InitialConditionSource=Input port
      settings: InputPortMap=u0,p4
  Delay78 : Delay  DelayLength=11  InitialConditionSource=Input port
      settings: InputPortMap=u0,p4
  Delay79 : Delay  DelayLength=12  InitialConditionSource=Input port
      settings: InputPortMap=u0,p4
  Delay80 : Delay  DelayLength=13  InitialConditionSource=Input port
      settings: InputPortMap=u0,p4
  Delay81 : Delay  DelayLength=14  InitialConditionSource=Input port
      settings: InputPortMap=u0,p4
  Delay82 : Delay  DelayLength=15  InitialConditionSource=Input port
      settings: InputPortMap=u0,p4
  Delay83 : Delay  DelayLength=16  InitialConditionSource=Input port
      settings: InputPortMap=u0,p4
  Delay84 : Delay  DelayLength=17  InitialConditionSource=Input port
      settings: InputPortMap=u0,p4
  Delay85 : Delay  DelayLength=18  InitialConditionSource=Input port
      settings: InputPortMap=u0,p4
  Delay86 : Delay  DelayLength=19  InitialConditionSource=Input port
      settings: InputPortMap=u0,p4
  Mux18 : Mux  Inputs=19
  delta_yaw_19 : Outport
  wires:
  Delay84/1 -> Mux18/17
  Delay72/1 -> Mux18/5
  Delay73/1 -> Mux18/6
  Delay78/1 -> Mux18/11
  Delay71/1 -> Mux18/4
  Delay68/1 -> Mux18/1
  Delay76/1 -> Mux18/9
  delta_yaw/1 -> Delay68/1, Delay68/2, Delay86/2, Delay86/1, Delay85/2, Delay85/1, Delay84/2, Delay84/1, Delay83/2, Delay83/1, Delay82/2, Delay82/1, Delay81/2, Delay81/1, Delay80/2, Delay80/1, Delay79/2, Delay79/1, Delay78/2, Delay78/1, Delay77/2, Delay77/1, Delay76/2, Delay76/1, Delay75/2, Delay75/1, Delay74/2, Delay74/1, Delay73/2, Delay73/1, Delay72/2, Delay72/1, Delay71/2, Delay71/1, Delay70/2, Delay70/1, Delay69/2, Delay69/1, Add78/1
  Delay81/1 -> Mux18/14
  Delay75/1 -> Mux18/8
  Delay80/1 -> Mux18/13
  Delay86/1 -> Mux18/19
  Delay82/1 -> Mux18/15
  Delay69/1 -> Mux18/2
  Delay70/1 -> Mux18/3
  Delay74/1 -> Mux18/7
  Mux18/1 -> Add78/2
  Delay77/1 -> Mux18/10
  Add78/1 -> delta_yaw_19/1
  Delay85/1 -> Mux18/18
  Delay79/1 -> Mux18/12
  Delay83/1 -> Mux18/16

== system acc_with_sensor/rolling_avg1 ==
  note: new_average = [ (sample_interval)/(sample_interval + time_constant) ] * (new_value - old_ave) + old_ave
  note: - (FK_TMR/TC)
      |                                    f  =  1  -  e
      |
      |       Where "f" is called the filter constant in the difference equation:
      |
      |                    new_average = f * new_value + (1 - f) * old_average
  note: Using the first two terms of the series expansion:
      |
      |                     x                     x2
      |                                e   =  1  +  x  +  --  + ......
      |                                           2!
      |
      |       Simplifying, the exponential "f" becomes:
      |
      |                  - (FK_TMR/TC)              1
      |           f  =  1  -  e                    =  1  -  -------------  =  . . .
      |                                                    (FK_TMR/TC)
      |                           e
      |
      |                              1                      1
      |          f  =  1  -  ---------------------------------  =    ------------------- .
      |                                  1 + (FK_TMR / TC)       1 + (TC / FK_TMR)
  new_value : Inport
  old_ave : Inport  Port=2
  delta_t : Inport  Port=3
  tc : Inport  Port=4
  Divide : Product  Inputs=*/
  IC : UnitDelay  Tag=struct('comment',struct('text','','placement',1),'logdata',struct('maxnumvals',inf,'plotchannels',[],'stepsize',0,'downsampling',1,'loggingmode',3,'channels',1),'output',struct('width',1,'name','$S_$B','unit','','type','Int16','offset',0,'max',NaN,'min',NaN,'freeze',1,'lsb',1,'arb',0,'class','default','address','','description','','autoscalingmode',1,'lowerheadroom',1,'upperheadroom',1,'headroomunit','bit','checkmin',0,'checkmax',0,'show',0,'initial','2'),'state',0,'dt','-1','date',731455.586925799)  InitialCondition=1  SampleTime=T  HasFrameUpgradeWarning=on
  Interval Test : simulink/Logic and Bit Operations/Interval Test  IntervalClosedRight=on  uplimit=0.00001  IntervalClosedLeft=on  lowlimit=-0.00001  OutDataTypeStr=boolean
  Logical Operator : Logic  Operator=NOT  AllPortsSameDT=off  OutDataTypeStr=boolean
  Product_tmp1 : Product  Tag=struct('comment',struct('text','','placement',1),'logdata',struct('maxnumvals',inf,'plotchannels',[],'stepsize',0,'downsampling',1,'loggingmode',3,'channels',1),'output',struct('width',1,'name','$S_$B','unit','','type','Int32Bin15','offset',0,'max',65535,'min',-65536,'freeze',1,'lsb',2^-15,'arb',0,'class','default','address','','description','','autoscalingmode',1,'lowerheadroom',1,'upperheadroom',1,'headroomunit','bit','checkmin',0,'checkmax',0,'show',0),'inputs','**','exceptionhandling',1,'date',731455.58640515)  Inputs=**  InputSameDT=on  RndMeth=Zero  OutDataTypeStr=Inherit: Same as first input
  Sum : Sum  Tag=struct('comment',struct('text','','placement',1),'logdata',struct('maxnumvals',inf,'plotchannels',[],'stepsize',0,'downsampling',1,'loggingmode',3,'channels',1),'output',struct('width',1,'name','$S_$B','unit','','type','Int32Bin15','offset',0,'max',65535,'min',-65536,'freeze',1,'lsb',2^-15,'arb',0,'class','default','address','','description','','autoscalingmode',1,'lowerheadroom',1,'upperheadroom',1,'headroomunit','bit','checkmin',0,'checkmax',0,'show',0),'inputs','-+','date',731455.586330463)  Inputs=-+  InputSameDT=on  OutDataTypeStr=Inherit: Same as first input
  Sum1 : Sum  Tag=struct('comment',struct('text','','placement',1),'logdata',struct('maxnumvals',inf,'plotchannels',[],'stepsize',0,'downsampling',1,'loggingmode',3,'channels',1),'output',struct('width',1,'name','$S_$B','unit','','type','Int32Bin15','offset',0,'max',65535,'min',-65536,'freeze',1,'lsb',2^-15,'arb',0,'class','default','address','','description','','autoscalingmode',1,'lowerheadroom',1,'upperheadroom',1,'headroomunit','bit','checkmin',0,'checkmax',0,'show',0),'inputs','++','date',731455.58628235)  InputSameDT=on  OutDataTypeStr=Inherit: Same as first input
  Sum2 : Sum  Tag=struct('comment',struct('text','','placement',1),'logdata',struct('maxnumvals',inf,'plotchannels',[],'stepsize',0,'downsampling',1,'loggingmode',3,'channels',1),'output',struct('width',1,'name','$S_$B','unit','','type','Int32Bin15','offset',0,'max',65535,'min',-65536,'freeze',1,'lsb',2^-15,'arb',0,'class','default','address','','description','','autoscalingmode',1,'lowerheadroom',1,'upperheadroom',1,'headroomunit','bit','checkmin',0,'checkmax',0,'show',0),'inputs','++','date',731455.586506424)  InputSameDT=on  OutDataTypeStr=Inherit: Same as first input
  Switch : Switch  Criteria=u2 ~= 0
  Switch1 : Switch  Tag=struct('comment',struct('text','','placement',1),'logdata',struct('maxnumvals',inf,'plotchannels',[],'stepsize',0,'downsampling',1,'loggingmode',3,'channels',1),'output',struct('width',1,'name','$S_$B','unit','','type','Int32Bin15','offset',0,'max',65535,'min',-65536,'freeze',1,'lsb',2^-15,'arb',0,'class','default','address','','description','','autoscalingmode',1,'lowerheadroom',1,'upperheadroom',1,'headroomunit','bit','checkmin',0,'checkmax',0,'show',0),'threshold',struct('width',1,'name','$S_$B_threshold','unit','','type','Int16','offset',0,'max',NaN,'min',NaN,'freeze',1,'lsb',1,'arb',0,'class','default','address','','description','','value','1','scalar',0),'date',731455.58657044)  Threshold=0.5  InputSameDT=on
  zero : Constant  Tag=struct('comment',struct('text','','placement',1),'output',struct('width',1,'name','$S_$B','unit','','type','Int16','offset',0,'max',NaN,'min',NaN,'freeze',1,'lsb',1,'arb',0,'class','default','address','','description','','value','0','tolerance',1,'show',0),'date',731455.58675544)  Value=0  OutDataTypeStr=Inherit: Inherit via back propagation
  zero1 : Constant  Tag=struct('comment',struct('text','','placement',1),'output',struct('width',1,'name','$S_$B','unit','','type','Int16','offset',0,'max',NaN,'min',NaN,'freeze',1,'lsb',1,'arb',0,'class','default','address','','description','','value','0','tolerance',1,'show',0),'date',731455.58675544)  Value=0  OutDataTypeStr=Inherit: Inherit via back propagation
  new_ave : Outport
  wires:
  Switch/1 -> Sum2/2
  Product_tmp1/1 -> Divide/1
  [new_value] -> Switch1/1
  Sum2/1 -> Switch1/3  "new_ave"
  new_value/1 -> [new_value], Sum/2  "new_value"
  Switch1/1 -> new_ave/1  "new_ave"
  Sum/1 -> Product_tmp1/1
  tc/1 -> Sum1/2
  delta_t/1 -> Sum1/1, Product_tmp1/2  "delta_t"
  zero/1 -> IC/1
  old_ave/1 -> Sum/1, Sum2/1  "old_ave"
  Sum1/1 -> Interval Test/1, Divide/2
  zero1/1 -> Switch/3
  Interval Test/1 -> Logical Operator/1
  Divide/1 -> Switch/1
  Logical Operator/1 -> Switch/2
  IC/1 -> Switch1/2

== system acc_with_sensor/Camera/Subsystem6 ==
  mps : Inport
  deg : Inport  Port=2
  Xo : Inport  Port=3
  Yo : Inport  Port=4
  station : Inport  Port=5
  Ax_HV_mps2 : Inport  Port=6
  Camera_NEW : MATLAB Function  TreatAsAtomicUnit=on
  Constant4 : Constant  Value=0.1  SampleTime=T
  Demux14 : Demux
  Subsystem16 : Subsystem
  Subsystem9 : Subsystem
  Terminator1 : Terminator  Commented=on
  Terminator2 : Terminator  Commented=on
  Terminator3 : Terminator  Commented=on
  LeftDis : Outport
  wires:
  mps/1 -> Camera_NEW/1(ux_mps), [Vx_HV_mps]
  [C2] -> Subsystem16/3("C2 ")
  [C1] -> Subsystem16/2(C1)
  [C0] -> Subsystem16/1(C0)
  [C3] -> Subsystem16/4(C3)
  Subsystem16/1(LeftDis) -> LeftDis/1
  Ax_HV_mps2/1 -> Subsystem16/6(Ax_HV_mps2)
  [Vx_HV_mps] -> Subsystem16/5(VehSpd_mps)
  Demux14/2 -> [C1]
  Demux14/4 -> [C3]
  Demux14/1 -> [C0]
  Demux14/3 -> [C2]
  Camera_NEW/4(C) -> Demux14/1
  station/1 -> Camera_NEW/5(station)
  Yo/1 -> Camera_NEW/4(Yo)
  deg/1 -> Camera_NEW/2(phi_deg)
  Xo/1 -> Camera_NEW/3(Xo)
  Subsystem9/3(Y_path) -> Camera_NEW/9(Y_path)
  Constant4/1 -> Camera_NEW/6(Ts_MPC)
  Subsystem9/2(s_path) -> Camera_NEW/8(s_path)
  Camera_NEW/3(Heading_ref) -> Terminator2/1
  Camera_NEW/1(x_ref) -> Terminator1/1
  Camera_NEW/2(y_ref) -> Terminator3/1  "yref"
  Subsystem9/1(X_path) -> Camera_NEW/7(X_path)

== system acc_with_sensor/Cut-in strategy/Subsystem8 ==
  TTC : Inport
  Mode : Inport  Port=2
  Constant1 : Constant  Value=0
  Gain : Gain  Gain=5
  Switch : Switch  Criteria=u2 ~= 0
  tau : Outport
  wires:
  Constant1/1 -> Switch/3
  TTC/1 -> Gain/1
  Switch/1 -> tau/1
  Mode/1 -> Switch/2
  Gain/1 -> Switch/1

== system acc_with_sensor/Old_Relative_Dynamic/acceleration_apr1 ==
  acc_b : Inport
  Abs : Abs
  Constant1 : Constant  Value=0
  Switch : Switch  Criteria=u2 > Threshold  Threshold=0.01
  acc_a : Outport  VectorParamsAs1DForOutWhenUnconnected=off
  wires:
  Switch/1 -> acc_a/1
  acc_b/1 -> Abs/1, Switch/1
  Constant1/1 -> Switch/3
  Abs/1 -> Switch/2

== system acc_with_sensor/Old_Relative_Dynamic/acceleration_apr4 ==
  acc_b : Inport
  Abs : Abs
  Constant1 : Constant  Value=0
  Switch : Switch  Criteria=u2 > Threshold  Threshold=0.01
  acc_a : Outport  VectorParamsAs1DForOutWhenUnconnected=off
  wires:
  Abs/1 -> Switch/2
  Constant1/1 -> Switch/3
  acc_b/1 -> Switch/1, Abs/1
  Switch/1 -> acc_a/1
